simulink model "m2_rayl2"  (R2018a)
settings: Solver=VariableStepAuto  StartTime=0.0  StopTime=30  RelTol=1e-3
undefined symbols (not defined in the file or in its folder): doppler
libraries: commutil2 x5, commdigbbndpm3 x2, commseqgen3 x2, commrandsrc3 x1, commsink2 x1, commchan3 x1
settings Model: Creator=acer  LastModifiedBy=12053

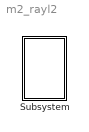
== system m2_rayl2 ==
  Subsystem : Subsystem  mask{Parameter1=0}

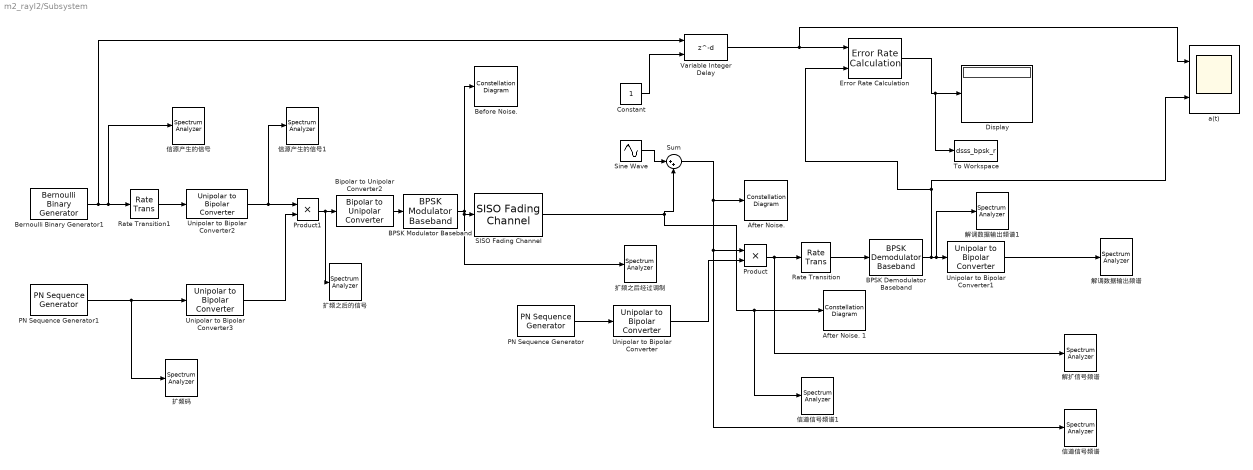
== system m2_rayl2/Subsystem ==
  "After Noise. " : ConstellationDiagram
  After Noise. 1 : ConstellationDiagram
  BPSK Demodulator Baseband : commdigbbndpm3/BPSK Demodulator Baseband  DecType=Hard decision  VarSource=Dialog  Variance=1  Ph=0  outDtype=Inherit via internal rule  derotateFactorWordLen=16  derotateFactorDataTypeStr=Inherit: Same word length as input  derotateFactorLastDataTypeStr=Inherit: Same word length as input
  BPSK Modulator Baseband : commdigbbndpm3/BPSK Modulator Baseband  Ph=0  outDtype=double  outWordLen=16  outUDDataType=sfix(16)  outFracLenMode=Best precision  outFracLen=15  outDataTypeStr=double  outLastDataTypeStr=double
  Before Noise. : ConstellationDiagram
  Bernoulli Binary Generator1 : commrandsrc3/Bernoulli Binary Generator  ProbabilityOfZero=0.5  SeedSource=Parameter  Seed=63  SampleTime=0.01  SamplesPerFrame=100  OutputDataType=double  SimulateUsing=Interpreted execution
  Bipolar to Unipolar Converter2 : commutil2/Bipolar to Unipolar Converter  M=2  polarity=Positive  dataType=Inherit via internal rule
      settings: SourceProductName=Communications System Toolbox  SourceProductBaseCode=CM
  Constant : Constant
  Display : Display
  Error Rate Calculation : commsink2/Error Rate Calculation  N=0  st_delay=0  cp_mode=Entire frame  subframe=[]  PMode=Port  WsName=ErrorRate  RsMode2=off  stop=off  numErr=100  maxBits=1e6
  PN Sequence Generator : commseqgen3/PN Sequence Generator  poly='z^6 + z + 1'  ini_sta=[0 0 0 0 0 1]  outBitMaskSource=Dialog parameter  shift=0  outVarSiz=off  maxOutSizeMode=Dialog parameter  maxOutSize=[10 1]  Ts=1/2000  sampPerFrame=1  reset=off  bitPackedOutputs=off  outDataType=double  numPackedBits=8  bitPackDataSigned=off  bitPackedOutDType=double
      settings: SourceProductName=Communications System Toolbox
  PN Sequence Generator1 : commseqgen3/PN Sequence Generator  poly='z^6 + z + 1'  ini_sta=[0 0 0 0 0 1]  outBitMaskSource=Dialog parameter  shift=0  outVarSiz=off  maxOutSizeMode=Dialog parameter  maxOutSize=[10 1]  Ts=1/2000  sampPerFrame=1  reset=off  bitPackedOutputs=off  outDataType=double  numPackedBits=8  bitPackDataSigned=off  bitPackedOutDType=double
      settings: SourceProductName=Communications System Toolbox
  Product : Product
  Product1 : Product
  Rate Transition : RateTransition  InitialCondition=1  OutPortSampleTime=1
  Rate Transition1 : RateTransition  Deterministic=off  OutPortSampleTime=1/2000
  SISO Fading Channel : commchan3/SISO Fading Channel  InheritSampleRate=on  SampleRate=100  PathDelays=[2e-6]  AveragePathGains=[-5]  NormalizePathGains=on  FadingDistribution=Rayleigh  KFactor=3  DirectPathDopplerShift=0  DirectPathInitialPhase=0  MaximumDopplerShift=100  DopplerSpectrum=doppler('Jakes')  ChannelInterpolationMethod=Polyphase  RandomStream=mt19937ar with seed  RandomNumGenerator=mt19937ar  Seed=12345  PathGainsOutputPort=off  ChannelFilterDelayOutputPort=off  SimulateUsing=Interpreted execution  Visualization=Off  PathsForDopplerDisplay=1  SamplesToDisplay=25%
      settings: SourceProductName=Communications System Toolbox
  Sine Wave : Sin  Frequency=300  SampleTime=1/2000
  Sum : Sum  Inputs=|++
  To Workspace : ToWorkspace  VariableName=dsss_bpsk_r  SampleTime=-1
      settings: Save2DSignal=2-D array (concatenate along first dimension)
  Unipolar to Bipolar Converter{,1..3} (4 alike) : commutil2/Unipolar to Bipolar Converter  M=2  polarity=Positive  dataType=Inherit via internal rule
      settings: SourceProductName=Communications System Toolbox
  Variable Integer Delay : Delay  DelayLengthSource=Input port
      settings: InputPortMap=u0,p1
  a(t) : Scope  NumInputPorts=2
  信源产生的信号 : SpectrumAnalyzer
  信源产生的信号1 : SpectrumAnalyzer
  信道信号频谱 : SpectrumAnalyzer
  信道信号频谱1 : SpectrumAnalyzer
  扩频之后的信号 : SpectrumAnalyzer
  扩频之后经过调制 : SpectrumAnalyzer
  扩频码 : SpectrumAnalyzer
  解扩信号频谱 : SpectrumAnalyzer
  解调数据输出频谱 : SpectrumAnalyzer
  解调数据输出频谱1 : SpectrumAnalyzer
  wires:
  Sine Wave/1 -> Sum/1
  PN Sequence Generator/1 -> Unipolar to Bipolar Converter/1
  Unipolar to Bipolar Converter/1 -> Product/2
  Unipolar to Bipolar Converter1/1 -> 解调数据输出频谱/1
  BPSK Modulator Baseband/1 -> 扩频之后经过调制/1, SISO Fading Channel/1, Before Noise./1
  SISO Fading Channel/1 -> Sum/2, 信道信号频谱1/1, After Noise. 1/1
  Product/1 -> 解扩信号频谱/1, Rate Transition/1
  Sum/1 -> "After Noise. "/1, 信道信号频谱/1, Product/1
  Bernoulli Binary Generator1/1 -> Variable Integer Delay/1, 信源产生的信号/1, Rate Transition1/1
  Error Rate Calculation/1 -> To Workspace/1, Display/1
  Rate Transition/1 -> BPSK Demodulator Baseband/1
  Variable Integer Delay/1 -> a(t)/1, Error Rate Calculation/1
  BPSK Demodulator Baseband/1 -> Error Rate Calculation/2, a(t)/2, 解调数据输出频谱1/1, Unipolar to Bipolar Converter1/1
  Constant/1 -> Variable Integer Delay/2
  Unipolar to Bipolar Converter2/1 -> 信源产生的信号1/1, Product1/1
  Rate Transition1/1 -> Unipolar to Bipolar Converter2/1
  PN Sequence Generator1/1 -> 扩频码/1, Unipolar to Bipolar Converter3/1
  Unipolar to Bipolar Converter3/1 -> Product1/2
  Product1/1 -> 扩频之后的信号/1, Bipolar to Unipolar Converter2/1
  Bipolar to Unipolar Converter2/1 -> BPSK Modulator Baseband/1
